simulink model "test"  (R2020a)
settings: Solver=FixedStepAuto  StartTime=0.0  StopTime=100  FixedStep=0.1  RelTol=1e-3
settings Model: Creator=KevinChan  LastModifiedBy=KevinChan

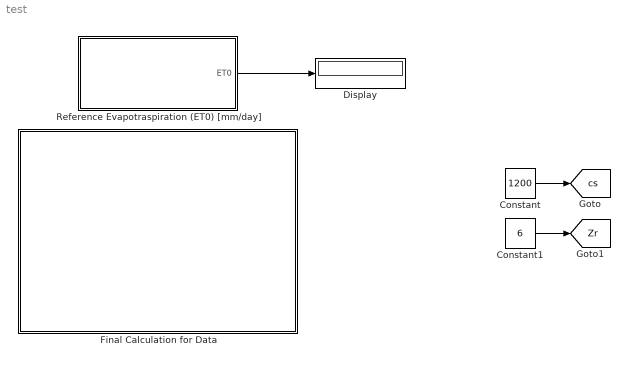
== system test ==
  " Final Calculation for Data" : Subsystem
  Constant : Constant  Value=1200
  Constant1 : Constant  Value=6
  Display : Display
  Reference Evapotraspiration (ET0) [mm/day] : Subsystem
  tag scope: Zr=global, cs=global
  wires:
  Reference Evapotraspiration (ET0) [mm/day]/1(ET0) -> Display/1
  Constant/1 -> [cs]
  Constant1/1 -> [Zr]

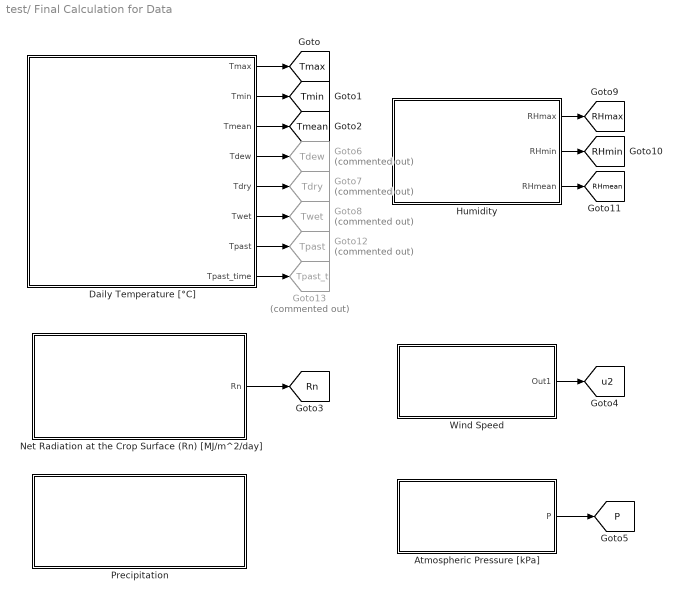
== system test/ Final Calculation for Data ==
  Atmospheric Pressure [kPa] : Subsystem
  Daily Temperature [°C] : Subsystem
  Goto12 : Goto  Commented=on  GotoTag=Tpast  TagVisibility=global
  Goto13 : Goto  Commented=on  GotoTag=Tpast_t  TagVisibility=global
  Goto6 : Goto  Commented=on  GotoTag=Tdew  TagVisibility=global
  Goto7 : Goto  Commented=on  GotoTag=Tdry  TagVisibility=global
  Goto8 : Goto  Commented=on  GotoTag=Twet  TagVisibility=global
  Humidity : Subsystem
  Net Radiation at the Crop Surface (Rn) [MJ/m^2/day] : Subsystem
  Precipitation : Subsystem
  Wind Speed : Subsystem
  tag scope: P=global, RHmax=global, RHmean=global, RHmin=global, Rn=global, Tmax=global, Tmean=global, Tmin=global, u2=global
  wires:
  Daily Temperature [°C]/1(Tmax) -> [Tmax]
  Daily Temperature [°C]/2(Tmin) -> [Tmin]
  Daily Temperature [°C]/3(Tmean) -> [Tmean]
  Net Radiation at the Crop Surface (Rn) [MJ/m^2/day]/1(Rn) -> [Rn]
  Wind Speed/1(Out1) -> [u2]
  Atmospheric Pressure [kPa]/1(P) -> [P]
  Daily Temperature [°C]/4(Tdew) -> Goto6/1
  Daily Temperature [°C]/5(Tdry) -> Goto7/1
  Daily Temperature [°C]/6(Twet) -> Goto8/1
  Humidity/1(RHmax) -> [RHmax]
  Humidity/3(RHmean) -> [RHmean]
  Humidity/2(RHmin) -> [RHmin]
  Daily Temperature [°C]/7(Tpast) -> Goto12/1
  Daily Temperature [°C]/8(Tpast_time) -> Goto13/1

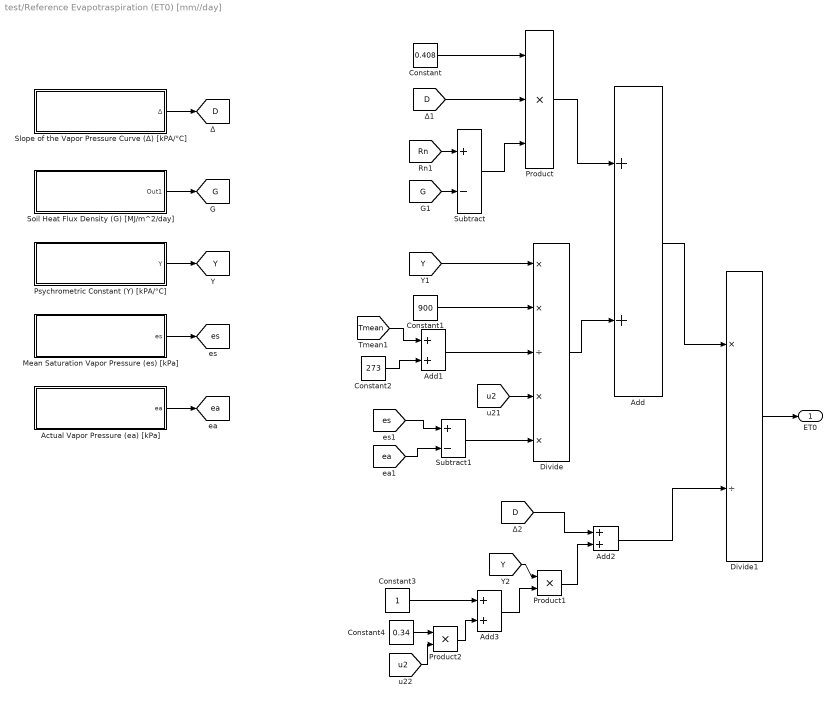
== system test/Reference Evapotraspiration (ET0) [mm//day] ==
  Actual Vapor Pressure (ea) [kPa] : Subsystem  mask{ea_choice=Derived from Relative Humidity Data (RHmean only), apsy_choice=0.000662 for ventilated (Asmann type) psychrometers, with an air movement of some 5 m/s}
      mask prompts: ea_choice "Select which method to derive:"; apsy_choice "Pick value for apsy:"
      mask init:
      | apsy = 0;
      | 
      | if apsy_choice == 1
      |     apsy = 0.000662;
      | elseif apsy_choice == 2
      |     apsy = 0.000800;
      | elseif apsy_choice == 3
      |     apsy = 0.001200;
      | end
      mask TypeOptions ea_choice: Derived from Dewpoint Temperature | Derived from Psyschrometirc Data | Derived from Relative Humidity Data (RHmax and RHmin) | Derived from Relative Humidity Data (RHmax only) | Derived from Relative Humidity Data (RHmean only)
      mask TypeOptions apsy_choice: 0.000662 for ventilated (Asmann type) psychrometers, with an air movement of some 5 m/s | 0.000800 for natural ventilated psychrometers (about 1 m/s) | 0.001200 for non-ventilated psychrometers installed indoors.
      mask DialogControl Control2 Prompt: There are 3 different ways to derive the actual vapor pressure. Depend on what data you have avaliable, pick the following choices. If you are picking relatitive humidity, beware of the following. When using equipment where errors in estimating RHmin can be large, or when RH data integrity are in doubt, then one should use only RHmax. In the absence of RHmax and RHmin, you can select to use RHmean.
      mask DialogControl Control3 Prompt: If you picked to use Psychrometric Data, select the folowing.
  Add{,1..3} (4 alike) : Sum
  Constant : Constant  Value=0.408
  Constant1 : Constant  Value=900
  Constant2 : Constant  Value=273
  Constant3 : Constant
  Constant4 : Constant  Value=0.34
  Divide : Product  Inputs=**/**
  Divide1 : Product  Inputs=*/
  "Mean Saturation Vapor Pressure (es) [kPa] " : Subsystem
  Product : Product  Inputs=3
  Product1 : Product
  Product2 : Product
  Psychrometric Constant (Y) [kPA/°C] : Subsystem
  Slope of the Vapor Pressure Curve (∆) [kPA/°C] : Subsystem
  Soil Heat Flux Density (G) [MJ/m^2/day] : Subsystem  mask{G_choice=For day and ten-day periods}
      mask prompts: G_choice "Select Time Step:"
      mask TypeOptions G_choice: For day and ten-day periods | For long periods
      mask DialogControl Control2 Prompt: For daily or weekly periods of time, soil heat flux density is small and can be ignored. A method to find G for long period of time is here, based on the idea that the soil temperature follows air temperature.
  Subtract : Sum  Inputs=+-
  Subtract1 : Sum  Inputs=+-
  ET0 : Outport
  tag scope: D=global, G=global, Y=global, ea=global, es=global
  wires:
  Divide1/1 -> ET0/1
  Constant/1 -> Product/1
  [D] -> Product/2
  [Rn] -> Subtract/1
  [G] -> Subtract/2
  Subtract/1 -> Product/3
  Product/1 -> Add/1
  Divide/1 -> Add/2
  Constant1/1 -> Divide/2
  [Tmean] -> Add1/1
  Constant2/1 -> Add1/2
  Add1/1 -> Divide/3
  Subtract1/1 -> Divide/5
  [es] -> Subtract1/1
  [ea] -> Subtract1/2
  Add/1 -> Divide1/1
  Add2/1 -> Divide1/2
  Product1/1 -> Add2/2
  Add3/1 -> Product1/2
  Constant3/1 -> Add3/1
  Product2/1 -> Add3/2
  Slope of the Vapor Pressure Curve (∆) [kPA/°C]/1(∆) -> [D]
  [D] -> Add2/1
  Soil Heat Flux Density (G) [MJ/m^2/day]/1(Out1) -> [G]
  Psychrometric Constant (Y) [kPA/°C]/1(Y) -> [Y]
  [Y] -> Divide/1
  [Y] -> Product1/1
  [u2] -> Divide/4
  [u2] -> Product2/2
  "Mean Saturation Vapor Pressure (es) [kPa] "/1(es) -> [es]
  Actual Vapor Pressure (ea) [kPa]/1(ea) -> [ea]
  Constant4/1 -> Product2/1

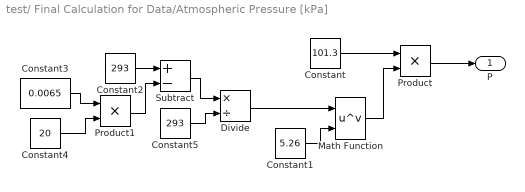
== system test/ Final Calculation for Data/Atmospheric Pressure [kPa] ==
  Constant : Constant  Value=101.3
  Constant1 : Constant  Value=5.26
  Constant2 : Constant  Value=293
  Constant3 : Constant  Value=0.0065
  Constant4 : Constant  Value=20
  Constant5 : Constant  Value=293
  Divide : Product  Inputs=*/
  Math Function : Math  Operator=pow  SaturateOnIntegerOverflow=on
  Product : Product
  Product1 : Product
  Subtract : Sum  Inputs=+-
  P : Outport
  wires:
  Product/1 -> P/1
  Constant/1 -> Product/1
  Math Function/1 -> Product/2
  Constant1/1 -> Math Function/2
  Divide/1 -> Math Function/1
  Subtract/1 -> Divide/1
  Constant2/1 -> Subtract/1
  Product1/1 -> Subtract/2
  Constant3/1 -> Product1/1
  Constant4/1 -> Product1/2
  Constant5/1 -> Divide/2

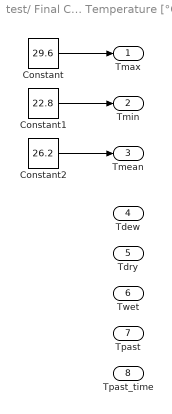
== system test/ Final Calculation for Data/Daily Temperature [°C] ==
  Constant : Constant  Value=29.6
  Constant1 : Constant  Value=22.8
  Constant2 : Constant  Value=26.2
  Tmax : Outport
  Tmin : Outport  Port=2
  Tmean : Outport  Port=3
  Tdew : Outport  Port=4
  Tdry : Outport  Port=5
  Twet : Outport  Port=6
  Tpast : Outport  Port=7
  Tpast_time : Outport  Port=8
  wires:
  Constant/1 -> Tmax/1
  Constant1/1 -> Tmin/1
  Constant2/1 -> Tmean/1

== system test/ Final Calculation for Data/Humidity ==
  Constant : Constant  Value=81
  Constant1 : Constant  Value=81
  Constant2 : Constant  Value=81
  RHmax : Outport
  RHmin : Outport  Port=2
  RHmean : Outport  Port=3
  wires:
  Constant/1 -> RHmax/1
  Constant1/1 -> RHmin/1
  Constant2/1 -> RHmean/1

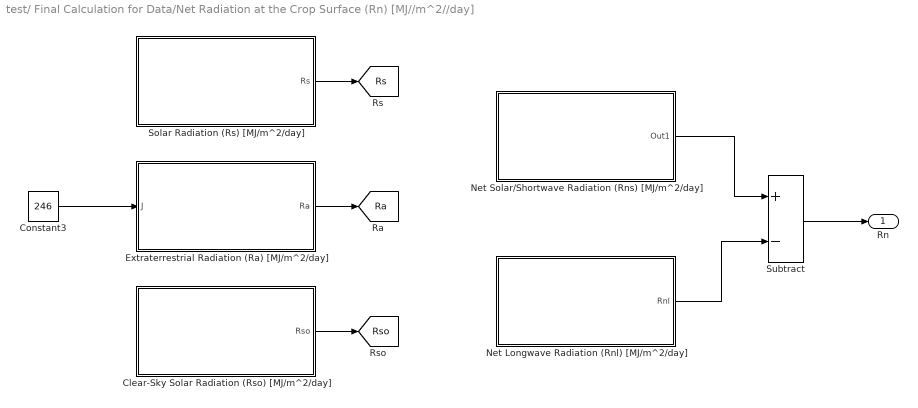
== system test/ Final Calculation for Data/Net Radiation at the Crop Surface (Rn) [MJ//m^2//day] ==
  Clear-Sky Solar Radiation (Rso) [MJ/m^2/day] : Subsystem
  Constant3 : Constant  Value=246
  Extraterrestrial Radiation (Ra) [MJ/m^2/day] : Subsystem
  Net Longwave Radiation (Rnl) [MJ/m^2/day] : Subsystem
  Net Solar/Shortwave Radiation (Rns) [MJ/m^2/day] : Subsystem
  Solar Radiation (Rs) [MJ/m^2/day] : Subsystem  mask{Ac_Rs=AI Predicted Solar Radiation}
      mask prompts: Ac_Rs "How to calculate Solar Radiation? (Most to Least Accurate)"
      mask TypeOptions Ac_Rs: AI Predicted Solar Radiation | Angstrom Formula if AI_Rs not avaliable | Hargreaves Formula if AI_Rs and hour of daylight is not available
  Subtract : Sum  Inputs=+-
  Rn : Outport
  tag scope: Ra=global, Rs=global, Rso=global
  wires:
  Subtract/1 -> Rn/1
  Net Solar/Shortwave Radiation (Rns) [MJ/m^2/day]/1(Out1) -> Subtract/1
  Net Longwave Radiation (Rnl) [MJ/m^2/day]/1(Rnl) -> Subtract/2
  Solar Radiation (Rs) [MJ/m^2/day]/1(Rs) -> [Rs]
  Extraterrestrial Radiation (Ra) [MJ/m^2/day]/1(Ra) -> [Ra]
  Constant3/1 -> Extraterrestrial Radiation (Ra) [MJ/m^2/day]/1(J)
  Clear-Sky Solar Radiation (Rso) [MJ/m^2/day]/1(Rso) -> [Rso]

== system test/ Final Calculation for Data/Precipitation ==

== system test/ Final Calculation for Data/Wind Speed ==
  Constant : Constant  Value=6739.2
  Constant1 : Constant  Value=2
  Wind Speed measured at 2m height (u2) [m/s] : Subsystem
  Out1 : Outport
  wires:
  Wind Speed measured at 2m height (u2) [m/s]/1(u2) -> Out1/1
  Constant1/1 -> Wind Speed measured at 2m height (u2) [m/s]/2(z)
  Constant/1 -> Wind Speed measured at 2m height (u2) [m/s]/1(uz)

== system test/Reference Evapotraspiration (ET0) [mm//day]/Actual Vapor Pressure (ea) [kPa] ==
  Constant : Constant  Value=ea_choice
  Derived from Dewpoint Temperature : Subsystem
  Derived from Psychrometric Data : Subsystem
  Derived from RHmax & RHmin : Subsystem
  Derived from RHmax only : Subsystem
  Derived from RHmean only : Subsystem
  Index Vector : MultiPortSwitch  Inputs=5
  ea : Outport
  wires:
  Derived from Dewpoint Temperature/1(Out1) -> Index Vector/2
  Index Vector/1 -> ea/1
  Constant/1 -> Index Vector/1
  Derived from Psychrometric Data/1(Out1) -> Index Vector/3
  Derived from RHmean only/1(Out1) -> Index Vector/6
  Derived from RHmax only/1(Out1) -> Index Vector/5
  Derived from RHmax & RHmin/1(Out1) -> Index Vector/4

== system test/Reference Evapotraspiration (ET0) [mm//day]/Mean Saturation Vapor Pressure (es) [kPa]  ==
  Add2 : Sum
  Constant6 : Constant  Value=2
  Divide2 : Product  Inputs=*/
  Saturation Vapor Pressure (eo) : Subsystem
  Saturation Vapor Pressure (eo) 2 : Subsystem
  es : Outport
  wires:
  Add2/1 -> Divide2/1
  Divide2/1 -> es/1
  Constant6/1 -> Divide2/2
  [Tmax] -> Saturation Vapor Pressure (eo)/1(In1)
  Saturation Vapor Pressure (eo)/1(Out1) -> Add2/1
  [Tmin] -> Saturation Vapor Pressure (eo) 2/1(In1)
  Saturation Vapor Pressure (eo) 2/1(Out1) -> Add2/2

== system test/Reference Evapotraspiration (ET0) [mm//day]/Psychrometric Constant (Y) [kPA//°C] ==
  Divide : Product  Inputs=**//
  Latent Heat of Vaporization (l) [MJ/kg] : Subsystem
  Ratio Molecular Weight of Water Vapour/Dry Air (e) : Constant  Value=0.622
  "Specific Heat at Constant Pressure (cp) [MJ/kg/°C] " : Constant  Value=0.001013
  Y : Outport
  wires:
  Divide/1 -> Y/1
  "Specific Heat at Constant Pressure (cp) [MJ/kg/°C] "/1 -> Divide/1
  Latent Heat of Vaporization (l) [MJ/kg]/1(l) -> Divide/4
  [P] -> Divide/2
  Ratio Molecular Weight of Water Vapour/Dry Air (e)/1 -> Divide/3

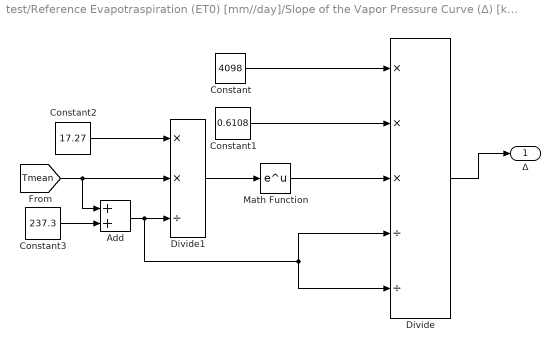
== system test/Reference Evapotraspiration (ET0) [mm//day]/Slope of the Vapor Pressure Curve (∆) [kPA//°C] ==
  Add : Sum
  Constant : Constant  Value=4098
  Constant1 : Constant  Value=0.6108
  Constant2 : Constant  Value=17.27
  Constant3 : Constant  Value=237.3
  Divide : Product  Inputs=***//
  Divide1 : Product  Inputs=**/
  Math Function : Math  SaturateOnIntegerOverflow=on
  ∆ : Outport
  wires:
  Divide/1 -> ∆/1
  Constant/1 -> Divide/1
  Constant1/1 -> Divide/2
  Math Function/1 -> Divide/3
  Divide1/1 -> Math Function/1
  [Tmean] -> Add/1, Divide1/2
  Constant2/1 -> Divide1/1
  Add/1 -> Divide/5, Divide/4, Divide1/3
  Constant3/1 -> Add/2

== system test/Reference Evapotraspiration (ET0) [mm//day]/Soil Heat Flux Density (G) [MJ//m^2//day] ==
  Constant : Constant  Value=G_choice
  For day and ten-day peroids : Constant  Value=0
  Index Vector : MultiPortSwitch  Inputs=2
  Long Time Steps : Subsystem
  Out1 : Outport
  wires:
  Long Time Steps/1(Out1) -> Index Vector/3
  For day and ten-day peroids/1 -> Index Vector/2
  Constant/1 -> Index Vector/1
  Index Vector/1 -> Out1/1

== system test/ Final Calculation for Data/Net Radiation at the Crop Surface (Rn) [MJ//m^2//day]/Clear-Sky Solar Radiation (Rso) [MJ//m^2//day] ==
  Add : Sum
  Constant : Constant  Value=0.75
  Constant1 : Constant  Value=0.00002
  Constant2 : Constant  Value=20
  Product : Product
  Product1 : Product
  Rso : Outport
  wires:
  Product/1 -> Rso/1
  [Ra] -> Product/2
  Add/1 -> Product/1
  Constant/1 -> Add/1
  Product1/1 -> Add/2
  Constant2/1 -> Product1/2
  Constant1/1 -> Product1/1

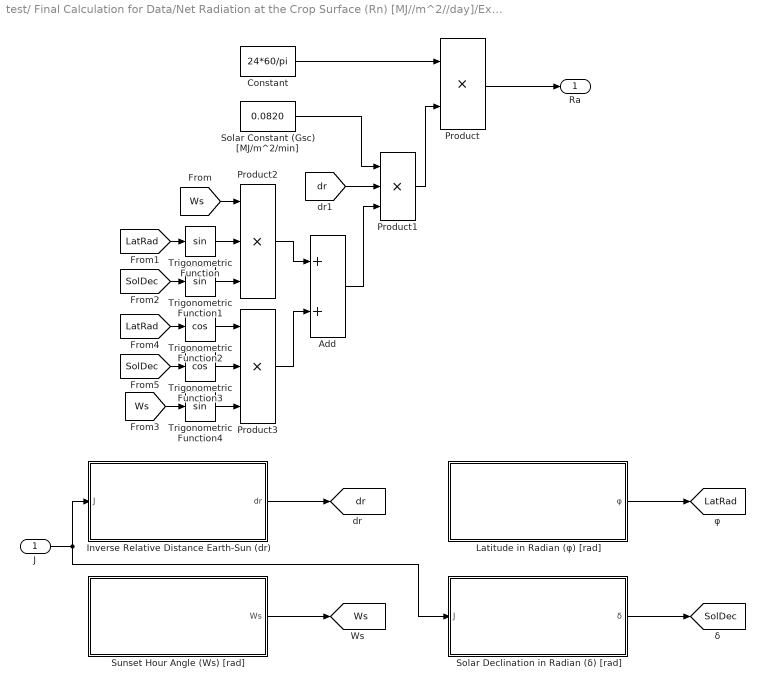
== system test/ Final Calculation for Data/Net Radiation at the Crop Surface (Rn) [MJ//m^2//day]/Extraterrestrial Radiation (Ra) [MJ//m^2//day] ==
  J : Inport
  Add : Sum
  Constant : Constant  Value=24*60/pi
  Inverse Relative Distance Earth-Sun (dr) : Subsystem
  Latitude in Radian (φ) [rad] : Subsystem
  Product : Product
  Product1 : Product  Inputs=3
  Product2 : Product  Inputs=3
  Product3 : Product  Inputs=3
  Solar Constant (Gsc) [MJ/m^2/min] : Constant  Value=0.0820
  Solar Declination in Radian (δ) [rad] : Subsystem
  Sunset Hour Angle (Ws) [rad] : Subsystem
  Trigonometric Function : Trigonometry
  Trigonometric Function1 : Trigonometry
  Trigonometric Function2 : Trigonometry  Operator=cos
  Trigonometric Function3 : Trigonometry  Operator=cos
  Trigonometric Function4 : Trigonometry
  Ra : Outport
  tag scope: LatRad=global, SolDec=global, Ws=global, dr=global
  wires:
  Constant/1 -> Product/1
  Product/1 -> Ra/1
  Product1/1 -> Product/2
  Solar Constant (Gsc) [MJ/m^2/min]/1 -> Product1/1
  Latitude in Radian (φ) [rad]/1(φ) -> [LatRad]
  Solar Declination in Radian (δ) [rad]/1(δ) -> [SolDec]
  Sunset Hour Angle (Ws) [rad]/1(Ws) -> [Ws]
  Inverse Relative Distance Earth-Sun (dr)/1(dr) -> [dr]
  [dr] -> Product1/2
  Trigonometric Function/1 -> Product2/2
  Trigonometric Function1/1 -> Product2/3
  [Ws] -> Product2/1
  [LatRad] -> Trigonometric Function/1
  [SolDec] -> Trigonometric Function1/1
  Product2/1 -> Add/1
  Add/1 -> Product1/3
  [SolDec] -> Trigonometric Function3/1
  [LatRad] -> Trigonometric Function2/1
  Product3/1 -> Add/2
  Trigonometric Function2/1 -> Product3/1
  Trigonometric Function3/1 -> Product3/2
  Trigonometric Function4/1 -> Product3/3
  [Ws] -> Trigonometric Function4/1
  J/1 -> Solar Declination in Radian (δ) [rad]/1(J), Inverse Relative Distance Earth-Sun (dr)/1(J)

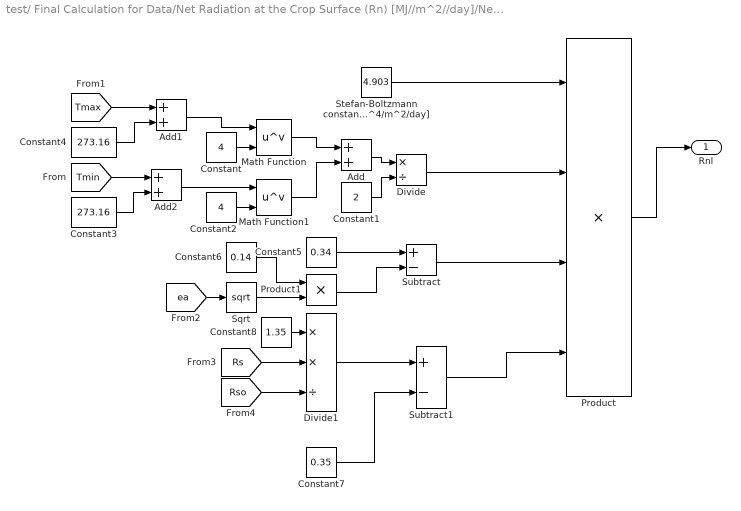
== system test/ Final Calculation for Data/Net Radiation at the Crop Surface (Rn) [MJ//m^2//day]/Net Longwave Radiation (Rnl) [MJ//m^2//day] ==
  Add : Sum
  Add1 : Sum
  Add2 : Sum
  Constant : Constant  Value=4
  Constant1 : Constant  Value=2
  Constant2 : Constant  Value=4
  Constant3 : Constant  Value=273.16
  Constant4 : Constant  Value=273.16
  Constant5 : Constant  Value=0.34
  Constant6 : Constant  Value=0.14
  Constant7 : Constant  Value=0.35
  Constant8 : Constant  Value=1.35
  Divide : Product  Inputs=*/
  Divide1 : Product  Inputs=**/
  Math Function : Math  Operator=pow  SaturateOnIntegerOverflow=on
  Math Function1 : Math  Operator=pow  SaturateOnIntegerOverflow=on
  Product : Product  Inputs=4
  Product1 : Product
  Sqrt : Sqrt  SaturateOnIntegerOverflow=on
  Stefan-Boltzmann constant (σ) [ 4.903 10^-9 MJ/K^4/m^2/day] : Constant  Value=4.903
  Subtract : Sum  Inputs=+-
  Subtract1 : Sum  Inputs=+-
  Rnl : Outport
  wires:
  Product/1 -> Rnl/1
  Stefan-Boltzmann constant (σ) [ 4.903 10^-9 MJ/K^4/m^2/day]/1 -> Product/1
  Constant/1 -> Math Function/2
  Math Function/1 -> Add/1
  Add/1 -> Divide/1
  Divide/1 -> Product/2
  Constant1/1 -> Divide/2
  Math Function1/1 -> Add/2
  Constant2/1 -> Math Function1/2
  Add1/1 -> Math Function/1
  Add2/1 -> Math Function1/1
  Constant3/1 -> Add2/2
  Constant4/1 -> Add1/2
  [Tmin] -> Add2/1
  [Tmax] -> Add1/1
  Subtract/1 -> Product/3
  Constant5/1 -> Subtract/1
  Product1/1 -> Subtract/2
  Constant6/1 -> Product1/1
  Sqrt/1 -> Product1/2
  [ea] -> Sqrt/1
  Subtract1/1 -> Product/4
  Divide1/1 -> Subtract1/1
  Constant7/1 -> Subtract1/2
  Constant8/1 -> Divide1/1
  [Rso] -> Divide1/3
  [Rs] -> Divide1/2

== system test/ Final Calculation for Data/Net Radiation at the Crop Surface (Rn) [MJ//m^2//day]/Net Solar//Shortwave Radiation (Rns) [MJ//m^2//day] ==
  Albedo or canopy reflection coefficient for the reference crop (G) : Subsystem
  Constant : Constant
  Product : Product
  Subtract : Sum  Inputs=+-
  Out1 : Outport
  wires:
  Product/1 -> Out1/1
  Constant/1 -> Subtract/1
  Albedo or canopy reflection coefficient for the reference crop (G)/1(Out1) -> Subtract/2
  Subtract/1 -> Product/1
  [Rs] -> Product/2

== system test/ Final Calculation for Data/Net Radiation at the Crop Surface (Rn) [MJ//m^2//day]/Solar Radiation (Rs) [MJ//m^2//day] ==
  Actual Duration of Sunlight (n) [hour] : Constant  Value=12
  Angstrom Formula if AI_Rs not avaliable : Subsystem
  Constant : Constant  Value=Ac_Rs
  Constant1 : Constant  Value=15.7
  Hargreaves Formula if AI_Rs and hour of daylight is not available : Subsystem  mask{kRs=0.16}
      mask prompts: kRs "Adjustment Coefficient"
      mask DialogControl Control2 Prompt: The square root of the temperature difference is closely related to the existing daily solar radiation in a given location. The adjustment coefficient kRs is empirical and differs for 'interior' or 'coastal' regions:
      mask DialogControl Control3 Prompt: · for 'interior' locations, where land mass dominates and air masses are not strongly influenced by a large water body, kRs @ 0.16;
      mask DialogControl Control4 Prompt: · for 'coastal' locations, situated on or adjacent to the coast of a large land mass and where air masses are influenced by a nearby water body, kRs @ 0.19.
  Index Vector : MultiPortSwitch
  Rs : Outport
  wires:
  Constant/1 -> Index Vector/1
  Constant1/1 -> Index Vector/2
  Angstrom Formula if AI_Rs not avaliable/1(Out1) -> Index Vector/3
  Index Vector/1 -> Rs/1
  Hargreaves Formula if AI_Rs and hour of daylight is not available/1(Rs) -> Index Vector/4
  Actual Duration of Sunlight (n) [hour]/1 -> Angstrom Formula if AI_Rs not avaliable/1(In1)

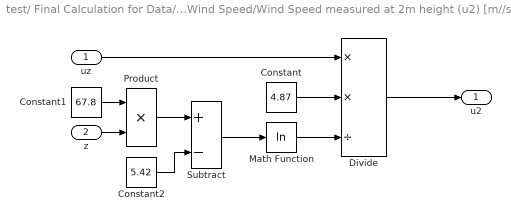
== system test/ Final Calculation for Data/Wind Speed/Wind Speed measured at 2m height (u2) [m//s] ==
  uz : Inport
  z : Inport  Port=2
  Constant : Constant  Value=4.87
  Constant1 : Constant  Value=67.8
  Constant2 : Constant  Value=5.42
  Divide : Product  Inputs=**/
  Math Function : Math  Operator=log  SaturateOnIntegerOverflow=on
  Product : Product
  Subtract : Sum  Inputs=+-
  u2 : Outport
  wires:
  uz/1 -> Divide/1
  Constant/1 -> Divide/2
  Math Function/1 -> Divide/3
  z/1 -> Product/2
  Constant1/1 -> Product/1
  Product/1 -> Subtract/1
  Subtract/1 -> Math Function/1
  Constant2/1 -> Subtract/2
  Divide/1 -> u2/1

== system test/Reference Evapotraspiration (ET0) [mm//day]/Actual Vapor Pressure (ea) [kPa]/Derived from Dewpoint Temperature ==
  Saturation Vapor Pressure (eo) : Subsystem
  Out1 : Outport
  wires:
  [Tdew] -> Saturation Vapor Pressure (eo)/1(In1)
  Saturation Vapor Pressure (eo)/1(Out1) -> Out1/1

== system test/Reference Evapotraspiration (ET0) [mm//day]/Actual Vapor Pressure (ea) [kPa]/Derived from Psychrometric Data ==
  Constant : Constant  Value=apsy
  Product : Product
  Product1 : Product
  Saturation Vapor Pressure (eo) : Subsystem
  Subtract : Sum  Inputs=+-
  Subtract1 : Sum  Inputs=+-
  Out1 : Outport
  wires:
  Subtract/1 -> Out1/1
  Saturation Vapor Pressure (eo)/1(Out1) -> Subtract/1
  [Twet] -> Subtract1/2, Saturation Vapor Pressure (eo)/1(In1)
  [Tdry] -> Subtract1/1
  Subtract1/1 -> Product/1
  Product/1 -> Subtract/2
  Product1/1 -> Product/2
  [P] -> Product1/2
  Constant/1 -> Product1/1

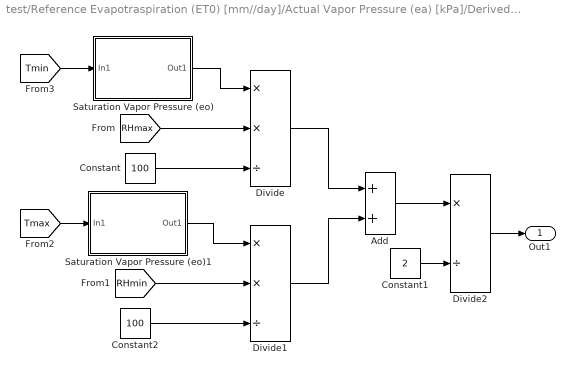
== system test/Reference Evapotraspiration (ET0) [mm//day]/Actual Vapor Pressure (ea) [kPa]/Derived from RHmax & RHmin ==
  Add : Sum
  Constant : Constant  Value=100
  Constant1 : Constant  Value=2
  Constant2 : Constant  Value=100
  Divide : Product  Inputs=**/
  Divide1 : Product  Inputs=**/
  Divide2 : Product  Inputs=*/
  Saturation Vapor Pressure (eo) : Subsystem
  Saturation Vapor Pressure (eo)1 : Subsystem
  Out1 : Outport
  wires:
  Divide2/1 -> Out1/1
  [Tmin] -> Saturation Vapor Pressure (eo)/1(In1)
  Saturation Vapor Pressure (eo)/1(Out1) -> Divide/1
  [RHmax] -> Divide/2
  Constant/1 -> Divide/3
  Divide/1 -> Add/1
  Divide1/1 -> Add/2
  Add/1 -> Divide2/1
  Constant1/1 -> Divide2/2
  Constant2/1 -> Divide1/3
  [RHmin] -> Divide1/2
  [Tmax] -> Saturation Vapor Pressure (eo)1/1(In1)
  Saturation Vapor Pressure (eo)1/1(Out1) -> Divide1/1

== system test/Reference Evapotraspiration (ET0) [mm//day]/Actual Vapor Pressure (ea) [kPa]/Derived from RHmax only ==
  Constant : Constant  Value=100
  Divide : Product  Inputs=**/
  Saturation Vapor Pressure (eo) : Subsystem
  Out1 : Outport
  wires:
  Constant/1 -> Divide/3
  [Tmin] -> Saturation Vapor Pressure (eo)/1(In1)
  [RHmax] -> Divide/2
  Saturation Vapor Pressure (eo)/1(Out1) -> Divide/1
  Divide/1 -> Out1/1

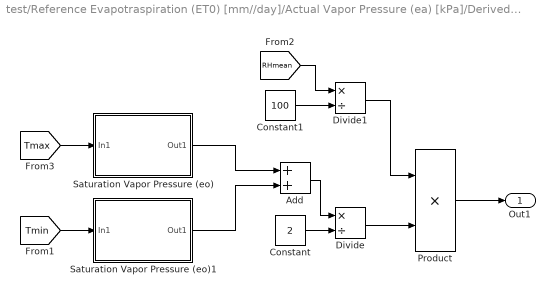
== system test/Reference Evapotraspiration (ET0) [mm//day]/Actual Vapor Pressure (ea) [kPa]/Derived from RHmean only ==
  Add : Sum
  Constant : Constant  Value=2
  Constant1 : Constant  Value=100
  Divide : Product  Inputs=*/
  Divide1 : Product  Inputs=*/
  Product : Product
  Saturation Vapor Pressure (eo) : Subsystem
  Saturation Vapor Pressure (eo)1 : Subsystem
  Out1 : Outport
  wires:
  [Tmax] -> Saturation Vapor Pressure (eo)/1(In1)
  Saturation Vapor Pressure (eo)/1(Out1) -> Add/1
  Saturation Vapor Pressure (eo)1/1(Out1) -> Add/2
  [Tmin] -> Saturation Vapor Pressure (eo)1/1(In1)
  Add/1 -> Divide/1
  Constant/1 -> Divide/2
  Divide/1 -> Product/2
  [RHmean] -> Divide1/1
  Constant1/1 -> Divide1/2
  Divide1/1 -> Product/1
  Product/1 -> Out1/1

== system test/Reference Evapotraspiration (ET0) [mm//day]/Mean Saturation Vapor Pressure (es) [kPa] /Saturation Vapor Pressure (eo) ==
  In1 : Inport
  Add : Sum
  Constant : Constant  Value=0.6108
  Constant1 : Constant  Value=17.27
  Constant2 : Constant  Value=237.3
  Divide : Product  Inputs=**/
  Math Function : Math  SaturateOnIntegerOverflow=on
  Product : Product
  Out1 : Outport
  wires:
  Product/1 -> Out1/1
  Constant1/1 -> Divide/1
  In1/1 -> Add/1, Divide/2
  Add/1 -> Divide/3
  Divide/1 -> Math Function/1
  Constant/1 -> Product/1
  Constant2/1 -> Add/2
  Math Function/1 -> Product/2

== system test/Reference Evapotraspiration (ET0) [mm//day]/Mean Saturation Vapor Pressure (es) [kPa] /Saturation Vapor Pressure (eo) 2 ==
  In1 : Inport
  Add1 : Sum
  Constant3 : Constant  Value=0.6108
  Constant4 : Constant  Value=17.27
  Constant5 : Constant  Value=237.3
  Divide1 : Product  Inputs=**/
  Math Function1 : Math  SaturateOnIntegerOverflow=on
  Product1 : Product
  Out1 : Outport
  wires:
  Math Function1/1 -> Product1/2
  Constant4/1 -> Divide1/1
  Add1/1 -> Divide1/3
  Constant3/1 -> Product1/1
  Divide1/1 -> Math Function1/1
  In1/1 -> Divide1/2, Add1/1
  Product1/1 -> Out1/1
  Constant5/1 -> Add1/2

== system test/Reference Evapotraspiration (ET0) [mm//day]/Psychrometric Constant (Y) [kPA//°C]/Latent Heat of Vaporization (l) [MJ//kg] ==
  "Latent Heat for an Air Temperature of about 20°C " : Constant  Value=2.45
  l : Outport
  wires:
  "Latent Heat for an Air Temperature of about 20°C "/1 -> l/1

== system test/Reference Evapotraspiration (ET0) [mm//day]/Soil Heat Flux Density (G) [MJ//m^2//day]/Long Time Steps ==
  Divide : Product  Inputs=**/*
  Subtract : Sum  Inputs=+-
  Out1 : Outport
  wires:
  [cs] -> Divide/1
  [Tmean] -> Subtract/1
  [Tpast] -> Subtract/2
  Subtract/1 -> Divide/2
  [Tpast_t] -> Divide/3
  [Zr] -> Divide/4
  Divide/1 -> Out1/1

== system test/ Final Calculation for Data/Net Radiation at the Crop Surface (Rn) [MJ//m^2//day]/Extraterrestrial Radiation (Ra) [MJ//m^2//day]/Inverse Relative Distance Earth-Sun (dr) ==
  J : Inport
  Add : Sum
  Constant : Constant
  Constant1 : Constant  Value=0.033
  Constant2 : Constant  Value=2*pi
  Constant3 : Constant  Value=365
  Divide : Product  Inputs=**/
  Product : Product
  Trigonometric Function : Trigonometry  Operator=cos
  dr : Outport
  wires:
  Add/1 -> dr/1
  Constant/1 -> Add/1
  Product/1 -> Add/2
  Constant1/1 -> Product/1
  Trigonometric Function/1 -> Product/2
  Divide/1 -> Trigonometric Function/1
  Constant2/1 -> Divide/1
  Constant3/1 -> Divide/3
  J/1 -> Divide/2

== system test/ Final Calculation for Data/Net Radiation at the Crop Surface (Rn) [MJ//m^2//day]/Extraterrestrial Radiation (Ra) [MJ//m^2//day]/Latitude in Radian (φ) [rad] ==
  Add : Sum
  Constant : Constant  Value=pi/180
  Constant1 : Constant  Value=60
  Constant2 : Constant  Value=-22
  Constant3 : Constant  Value=-54
  Divide : Product  Inputs=*/
  Product : Product
  φ : Outport
  wires:
  Constant/1 -> Product/1
  Add/1 -> Product/2
  Constant2/1 -> Add/1
  Constant3/1 -> Divide/1
  Constant1/1 -> Divide/2
  Divide/1 -> Add/2
  Product/1 -> φ/1

== system test/ Final Calculation for Data/Net Radiation at the Crop Surface (Rn) [MJ//m^2//day]/Extraterrestrial Radiation (Ra) [MJ//m^2//day]/Solar Declination in Radian (δ) [rad] ==
  J : Inport
  Constant : Constant  Value=365
  Constant1 : Constant  Value=0.409
  Constant2 : Constant  Value=2*pi
  Constant4 : Constant  Value=1.39
  Divide : Product  Inputs=**/
  Product : Product
  Subtract : Sum  Inputs=+-
  Trigonometric Function : Trigonometry
  δ : Outport
  wires:
  Constant/1 -> Divide/3
  Product/1 -> δ/1
  Trigonometric Function/1 -> Product/2
  J/1 -> Divide/2
  Constant2/1 -> Divide/1
  Constant1/1 -> Product/1
  Divide/1 -> Subtract/1
  Subtract/1 -> Trigonometric Function/1
  Constant4/1 -> Subtract/2

== system test/ Final Calculation for Data/Net Radiation at the Crop Surface (Rn) [MJ//m^2//day]/Extraterrestrial Radiation (Ra) [MJ//m^2//day]/Sunset Hour Angle (Ws) [rad] ==
  Constant : Constant  Value=-1
  Product : Product  Inputs=3
  Trigonometric Function : Trigonometry  Operator=acos
  Trigonometric Function1 : Trigonometry  Operator=tan
  Trigonometric Function2 : Trigonometry  Operator=tan
  Ws : Outport
  wires:
  Trigonometric Function/1 -> Ws/1
  Product/1 -> Trigonometric Function/1
  Constant/1 -> Product/1
  Trigonometric Function1/1 -> Product/2
  Trigonometric Function2/1 -> Product/3
  [LatRad] -> Trigonometric Function1/1
  [SolDec] -> Trigonometric Function2/1

== system test/ Final Calculation for Data/Net Radiation at the Crop Surface (Rn) [MJ//m^2//day]/Net Solar//Shortwave Radiation (Rns) [MJ//m^2//day]/Albedo or canopy reflection coefficient for the reference crop (G) ==
  Constant : Constant  Value=0.23
  Out1 : Outport
  wires:
  Constant/1 -> Out1/1

== system test/ Final Calculation for Data/Net Radiation at the Crop Surface (Rn) [MJ//m^2//day]/Solar Radiation (Rs) [MJ//m^2//day]/Angstrom Formula if AI_Rs not avaliable ==
  In1 : Inport
  Add : Sum
  Default as : Constant  Value=0.25
  Default bs : Constant  Value=0.50
  Divide : Product  Inputs=**/
  Maximum Daylight Hour (N) [hour] : Subsystem
  Product : Product
  Out1 : Outport
  wires:
  Default as/1 -> Add/1
  Default bs/1 -> Divide/1
  Divide/1 -> Add/2
  In1/1 -> Divide/2
  Add/1 -> Product/1
  Product/1 -> Out1/1
  [Ra] -> Product/2
  Maximum Daylight Hour (N) [hour]/1(N) -> Divide/3

== system test/ Final Calculation for Data/Net Radiation at the Crop Surface (Rn) [MJ//m^2//day]/Solar Radiation (Rs) [MJ//m^2//day]/Hargreaves Formula if AI_Rs and hour of daylight is not available ==
  Constant : Constant  Value=kRs
  Product : Product  Inputs=3
  Sqrt : Sqrt  SaturateOnIntegerOverflow=on
  Subtract : Sum  Inputs=+-
  Rs : Outport
  wires:
  Product/1 -> Rs/1
  Constant/1 -> Product/1
  [Ra] -> Product/3
  Sqrt/1 -> Product/2
  Subtract/1 -> Sqrt/1
  [Tmin] -> Subtract/2
  [Tmax] -> Subtract/1

== system test/Reference Evapotraspiration (ET0) [mm//day]/Actual Vapor Pressure (ea) [kPa]/Derived from Dewpoint Temperature/Saturation Vapor Pressure (eo) ==
  In1 : Inport
  Add : Sum
  Constant : Constant  Value=0.6108
  Constant1 : Constant  Value=17.27
  Constant2 : Constant  Value=237.3
  Divide : Product  Inputs=**/
  Math Function : Math  SaturateOnIntegerOverflow=on
  Product : Product
  Out1 : Outport
  wires:
  Product/1 -> Out1/1
  Constant1/1 -> Divide/1
  In1/1 -> Add/1, Divide/2
  Add/1 -> Divide/3
  Divide/1 -> Math Function/1
  Constant/1 -> Product/1
  Constant2/1 -> Add/2
  Math Function/1 -> Product/2

== system test/Reference Evapotraspiration (ET0) [mm//day]/Actual Vapor Pressure (ea) [kPa]/Derived from Psychrometric Data/Saturation Vapor Pressure (eo) ==
  In1 : Inport
  Add : Sum
  Constant : Constant  Value=0.6108
  Constant1 : Constant  Value=17.27
  Constant2 : Constant  Value=237.3
  Divide : Product  Inputs=**/
  Math Function : Math  SaturateOnIntegerOverflow=on
  Product : Product
  Out1 : Outport
  wires:
  Product/1 -> Out1/1
  Constant1/1 -> Divide/1
  In1/1 -> Add/1, Divide/2
  Add/1 -> Divide/3
  Divide/1 -> Math Function/1
  Constant/1 -> Product/1
  Constant2/1 -> Add/2
  Math Function/1 -> Product/2

== system test/Reference Evapotraspiration (ET0) [mm//day]/Actual Vapor Pressure (ea) [kPa]/Derived from RHmax & RHmin/Saturation Vapor Pressure (eo) ==
  In1 : Inport
  Add : Sum
  Constant : Constant  Value=0.6108
  Constant1 : Constant  Value=17.27
  Constant2 : Constant  Value=237.3
  Divide : Product  Inputs=**/
  Math Function : Math  SaturateOnIntegerOverflow=on
  Product : Product
  Out1 : Outport
  wires:
  Product/1 -> Out1/1
  Constant1/1 -> Divide/1
  In1/1 -> Add/1, Divide/2
  Add/1 -> Divide/3
  Divide/1 -> Math Function/1
  Constant/1 -> Product/1
  Constant2/1 -> Add/2
  Math Function/1 -> Product/2

== system test/Reference Evapotraspiration (ET0) [mm//day]/Actual Vapor Pressure (ea) [kPa]/Derived from RHmax & RHmin/Saturation Vapor Pressure (eo)1 ==
  In1 : Inport
  Add : Sum
  Constant : Constant  Value=0.6108
  Constant1 : Constant  Value=17.27
  Constant2 : Constant  Value=237.3
  Divide : Product  Inputs=**/
  Math Function : Math  SaturateOnIntegerOverflow=on
  Product : Product
  Out1 : Outport
  wires:
  Math Function/1 -> Product/2
  Constant2/1 -> Add/2
  Constant/1 -> Product/1
  Divide/1 -> Math Function/1
  Add/1 -> Divide/3
  In1/1 -> Divide/2, Add/1
  Constant1/1 -> Divide/1
  Product/1 -> Out1/1

== system test/Reference Evapotraspiration (ET0) [mm//day]/Actual Vapor Pressure (ea) [kPa]/Derived from RHmax only/Saturation Vapor Pressure (eo) ==
  In1 : Inport
  Add : Sum
  Constant : Constant  Value=0.6108
  Constant1 : Constant  Value=17.27
  Constant2 : Constant  Value=237.3
  Divide : Product  Inputs=**/
  Math Function : Math  SaturateOnIntegerOverflow=on
  Product : Product
  Out1 : Outport
  wires:
  Product/1 -> Out1/1
  Constant1/1 -> Divide/1
  In1/1 -> Add/1, Divide/2
  Add/1 -> Divide/3
  Divide/1 -> Math Function/1
  Constant/1 -> Product/1
  Constant2/1 -> Add/2
  Math Function/1 -> Product/2

== system test/Reference Evapotraspiration (ET0) [mm//day]/Actual Vapor Pressure (ea) [kPa]/Derived from RHmean only/Saturation Vapor Pressure (eo) ==
  In1 : Inport
  Add : Sum
  Constant : Constant  Value=0.6108
  Constant1 : Constant  Value=17.27
  Constant2 : Constant  Value=237.3
  Divide : Product  Inputs=**/
  Math Function : Math  SaturateOnIntegerOverflow=on
  Product : Product
  Out1 : Outport
  wires:
  Product/1 -> Out1/1
  Constant1/1 -> Divide/1
  In1/1 -> Add/1, Divide/2
  Add/1 -> Divide/3
  Divide/1 -> Math Function/1
  Constant/1 -> Product/1
  Constant2/1 -> Add/2
  Math Function/1 -> Product/2

== system test/Reference Evapotraspiration (ET0) [mm//day]/Actual Vapor Pressure (ea) [kPa]/Derived from RHmean only/Saturation Vapor Pressure (eo)1 ==
  In1 : Inport
  Add : Sum
  Constant : Constant  Value=0.6108
  Constant1 : Constant  Value=17.27
  Constant2 : Constant  Value=237.3
  Divide : Product  Inputs=**/
  Math Function : Math  SaturateOnIntegerOverflow=on
  Product : Product
  Out1 : Outport
  wires:
  Math Function/1 -> Product/2
  Constant2/1 -> Add/2
  Constant/1 -> Product/1
  Divide/1 -> Math Function/1
  Add/1 -> Divide/3
  In1/1 -> Divide/2, Add/1
  Constant1/1 -> Divide/1
  Product/1 -> Out1/1

== system test/ Final Calculation for Data/Net Radiation at the Crop Surface (Rn) [MJ//m^2//day]/Solar Radiation (Rs) [MJ//m^2//day]/Angstrom Formula if AI_Rs not avaliable/Maximum Daylight Hour (N) [hour] ==
  Constant : Constant  Value=24
  Constant1 : Constant  Value=pi
  Divide : Product  Inputs=**/
  N : Outport
  wires:
  Divide/1 -> N/1
  [Ws] -> Divide/2
  Constant/1 -> Divide/1
  Constant1/1 -> Divide/3
